simulink model "MotorCurrentEKF_"  (R2018a)
settings: Solver=VariableStepAuto  StartTime=0.0  StopTime=10.0  RelTol=1e-3
PreLoadFcn:
  | modelDir = fileparts(get_param(bdroot, 'FileName'));
  | addpath(fullfile(modelDir,'../Parameters'));
  | 
  | Parameters_Model
  | Parameters_Simulation
  | Parameters_Estimators
InitFcn:
  | Parameters_Model
  | Parameters_Simulation
  | Parameters_Estimators
undefined symbols (not defined in the file): Ke, L, P_init, X_init
settings Model: Creator=Thomas  LastModifiedBy=Thomas

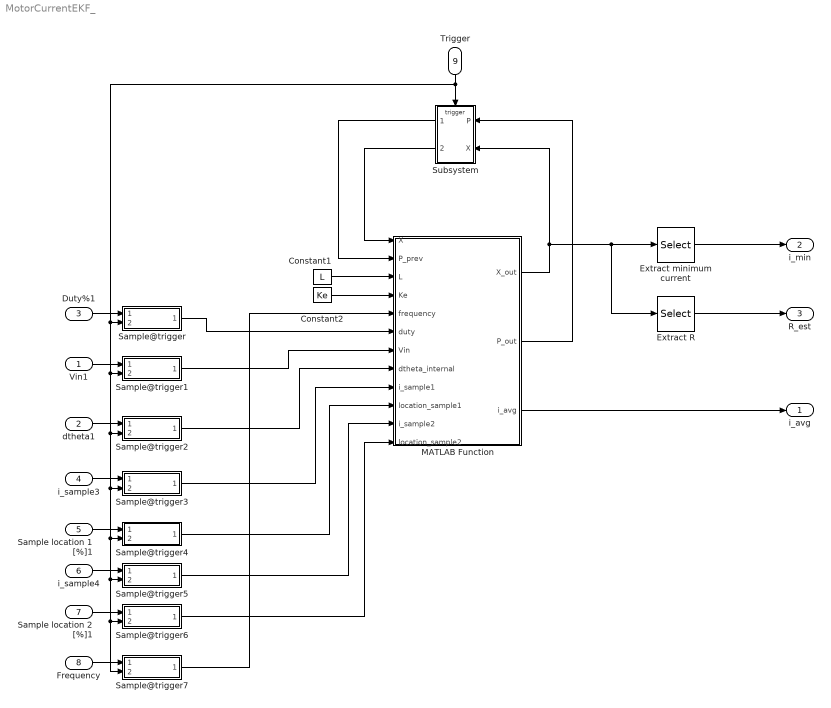
== system MotorCurrentEKF_ ==
  Vin1 : Inport  OutDataTypeStr=double
  dtheta1 : Inport  Port=2  OutDataTypeStr=double
  Duty%1 : Inport  Port=3  OutDataTypeStr=double
  i_sample3 : Inport  Port=4  OutDataTypeStr=double
  Sample location 1 [%]1 : Inport  Port=5  OutDataTypeStr=double
  i_sample4 : Inport  Port=6  OutDataTypeStr=double
  Sample location 2 [%]1 : Inport  Port=7  OutDataTypeStr=double
  Frequency : Inport  Port=8  OutDataTypeStr=double
  Trigger : Inport  Port=9  OutDataTypeStr=boolean
  Constant1 : Constant  Value=L
  Constant2 : Constant  Value=Ke
  Extract R : Selector  InputPortWidth=2  IndexOptions=Index vector (dialog)  Indices=[2]  OutputSizes=1
  Extract minimum current : Selector  InputPortWidth=2  IndexOptions=Index vector (dialog)  Indices=[1]  OutputSizes=1
  MATLAB Function : MATLAB Function  TreatAsAtomicUnit=on
  Sample@trigger : Subsystem
  Sample@trigger1 : Subsystem
  Sample@trigger2 : Subsystem
  Sample@trigger3 : Subsystem
  Sample@trigger4 : Subsystem
  Sample@trigger5 : Subsystem
  Sample@trigger6 : Subsystem
  Sample@trigger7 : Subsystem
  Subsystem : Subsystem
  i_avg : Outport
  i_min : Outport  Port=2
  R_est : Outport  Port=3
  wires:
  MATLAB Function/1(X_out) -> Subsystem/2(X), Extract R/1, Extract minimum current/1
  MATLAB Function/2(P_out) -> Subsystem/1(P)
  Subsystem/1(P_prev) -> MATLAB Function/2(P_prev)
  Subsystem/2(X_prev) -> MATLAB Function/1(X)
  Constant1/1 -> MATLAB Function/3(L)
  Constant2/1 -> MATLAB Function/4(Ke)
  MATLAB Function/3(i_avg) -> i_avg/1
  Extract minimum current/1 -> i_min/1
  Extract R/1 -> R_est/1
  Duty%1/1 -> Sample@trigger/1(Signal)
  Trigger/1 -> Sample@trigger1/2(Trigger), Sample@trigger2/2(Trigger), Sample@trigger3/2(Trigger), Sample@trigger4/2(Trigger), Sample@trigger7/2(Trigger), Sample@trigger6/2(Trigger), Sample@trigger5/2(Trigger), Sample@trigger/2(Trigger), Subsystem/Trigger
  Frequency/1 -> Sample@trigger7/1(Signal)
  Sample location 2 [%]1/1 -> Sample@trigger6/1(Signal)
  Vin1/1 -> Sample@trigger1/1(Signal)
  dtheta1/1 -> Sample@trigger2/1(Signal)
  Sample location 1 [%]1/1 -> Sample@trigger4/1(Signal)
  i_sample3/1 -> Sample@trigger3/1(Signal)
  i_sample4/1 -> Sample@trigger5/1(Signal)
  Sample@trigger/1(Sample) -> MATLAB Function/6(duty)
  Sample@trigger1/1(Sample) -> MATLAB Function/7(Vin)
  Sample@trigger2/1(Sample) -> MATLAB Function/8(dtheta_internal)
  Sample@trigger3/1(Sample) -> MATLAB Function/9(i_sample1)
  Sample@trigger4/1(Sample) -> MATLAB Function/10(location_sample1)
  Sample@trigger5/1(Sample) -> MATLAB Function/11(i_sample2)
  Sample@trigger6/1(Sample) -> MATLAB Function/12(location_sample2)
  Sample@trigger7/1(Sample) -> MATLAB Function/5(frequency)

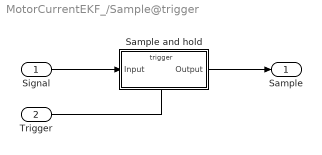
== system MotorCurrentEKF_/Sample@trigger ==
  Signal : Inport
  Trigger : Inport  Port=2
  Sample and hold : Subsystem
  Sample : Outport
  wires:
  Signal/1 -> Sample and hold/1(Input)
  Sample and hold/1(Output) -> Sample/1
  Trigger/1 -> Sample and hold/Trigger

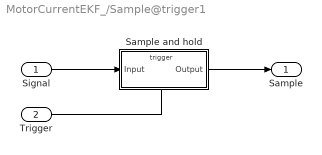
== system MotorCurrentEKF_/Sample@trigger1 ==
  Signal : Inport
  Trigger : Inport  Port=2
  Sample and hold : Subsystem
  Sample : Outport
  wires:
  Signal/1 -> Sample and hold/1(Input)
  Sample and hold/1(Output) -> Sample/1
  Trigger/1 -> Sample and hold/Trigger

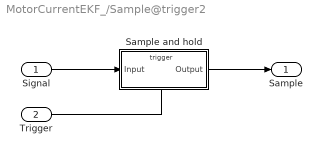
== system MotorCurrentEKF_/Sample@trigger2 ==
  Signal : Inport
  Trigger : Inport  Port=2
  Sample and hold : Subsystem
  Sample : Outport
  wires:
  Signal/1 -> Sample and hold/1(Input)
  Sample and hold/1(Output) -> Sample/1
  Trigger/1 -> Sample and hold/Trigger

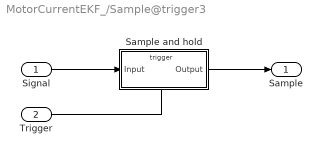
== system MotorCurrentEKF_/Sample@trigger3 ==
  Signal : Inport
  Trigger : Inport  Port=2
  Sample and hold : Subsystem
  Sample : Outport
  wires:
  Signal/1 -> Sample and hold/1(Input)
  Sample and hold/1(Output) -> Sample/1
  Trigger/1 -> Sample and hold/Trigger

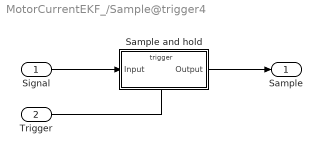
== system MotorCurrentEKF_/Sample@trigger4 ==
  Signal : Inport
  Trigger : Inport  Port=2
  Sample and hold : Subsystem
  Sample : Outport
  wires:
  Signal/1 -> Sample and hold/1(Input)
  Sample and hold/1(Output) -> Sample/1
  Trigger/1 -> Sample and hold/Trigger

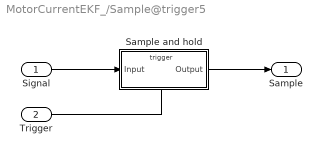
== system MotorCurrentEKF_/Sample@trigger5 ==
  Signal : Inport
  Trigger : Inport  Port=2
  Sample and hold : Subsystem
  Sample : Outport
  wires:
  Signal/1 -> Sample and hold/1(Input)
  Sample and hold/1(Output) -> Sample/1
  Trigger/1 -> Sample and hold/Trigger

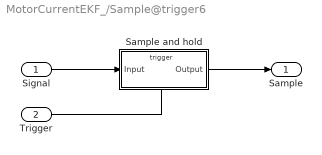
== system MotorCurrentEKF_/Sample@trigger6 ==
  Signal : Inport
  Trigger : Inport  Port=2
  Sample and hold : Subsystem
  Sample : Outport
  wires:
  Signal/1 -> Sample and hold/1(Input)
  Sample and hold/1(Output) -> Sample/1
  Trigger/1 -> Sample and hold/Trigger

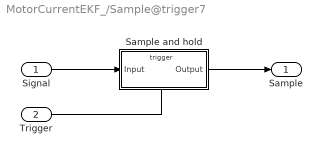
== system MotorCurrentEKF_/Sample@trigger7 ==
  Signal : Inport
  Trigger : Inport  Port=2
  Sample and hold : Subsystem
  Sample : Outport
  wires:
  Signal/1 -> Sample and hold/1(Input)
  Sample and hold/1(Output) -> Sample/1
  Trigger/1 -> Sample and hold/Trigger

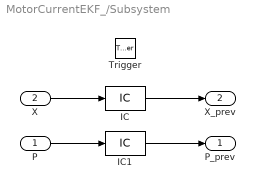
== system MotorCurrentEKF_/Subsystem ==
  P : Inport  LatchByDelayingOutsideSignal=on
  X : Inport  Port=2  LatchByDelayingOutsideSignal=on
  Trigger : TriggerPort  VariantControl=Variant  PortDimensions=1
  IC : InitialCondition  Value=X_init
  IC1 : InitialCondition  Value=P_init
  P_prev : Outport
  X_prev : Outport  Port=2
  wires:
  X/1 -> IC/1
  P/1 -> IC1/1
  IC/1 -> X_prev/1
  IC1/1 -> P_prev/1

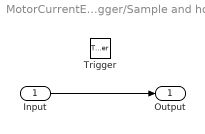
== system MotorCurrentEKF_/Sample@trigger/Sample and hold ==
  Input : Inport
  Trigger : TriggerPort  VariantControl=Variant  PortDimensions=1
  Output : Outport
  wires:
  Input/1 -> Output/1

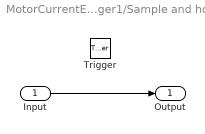
== system MotorCurrentEKF_/Sample@trigger1/Sample and hold ==
  Input : Inport
  Trigger : TriggerPort  VariantControl=Variant  PortDimensions=1
  Output : Outport
  wires:
  Input/1 -> Output/1

== system MotorCurrentEKF_/Sample@trigger2/Sample and hold ==
  Input : Inport
  Trigger : TriggerPort  VariantControl=Variant  PortDimensions=1
  Output : Outport
  wires:
  Input/1 -> Output/1

== system MotorCurrentEKF_/Sample@trigger3/Sample and hold ==
  Input : Inport
  Trigger : TriggerPort  VariantControl=Variant  PortDimensions=1
  Output : Outport
  wires:
  Input/1 -> Output/1

== system MotorCurrentEKF_/Sample@trigger4/Sample and hold ==
  Input : Inport
  Trigger : TriggerPort  VariantControl=Variant  PortDimensions=1
  Output : Outport
  wires:
  Input/1 -> Output/1

== system MotorCurrentEKF_/Sample@trigger5/Sample and hold ==
  Input : Inport
  Trigger : TriggerPort  VariantControl=Variant  PortDimensions=1
  Output : Outport
  wires:
  Input/1 -> Output/1

== system MotorCurrentEKF_/Sample@trigger6/Sample and hold ==
  Input : Inport
  Trigger : TriggerPort  VariantControl=Variant  PortDimensions=1
  Output : Outport
  wires:
  Input/1 -> Output/1

== system MotorCurrentEKF_/Sample@trigger7/Sample and hold ==
  Input : Inport
  Trigger : TriggerPort  VariantControl=Variant  PortDimensions=1
  Output : Outport
  wires:
  Input/1 -> Output/1

== matlab function MotorCurrentEKF_/MATLAB Function ==
  data: X input; X_out output; P_prev input; L input; Ke input; frequency input; duty input; Vin input; dtheta_internal input; i_sample1 input; location_sample1 input; P_out output; i_avg output; i_sample2 input; location_sample2 input
function [X_out, P_out, i_avg] = MotorCurrentEKF_(X, P_prev, ...
    L, Ke, ... % constants/parameters
    frequency, duty, Vin, dtheta_internal, ... % inputs (u)
    i_sample1, location_sample1, ...
    i_sample2, location_sample2)  % measurements (z)

%     [X_out, P_out] = MotorCurrentEKF(X, P_prev, ...
%         R, L, Ke, ... % constants/parameters
%         frequency, duty, Vin, dtheta_internal, ... % inputs (u)
%         i_meas, adc_sample_time);  % measurements (z)

    [X_out, P_out, i_avg] = MotorCurrentEKF7(X, P_prev, ...
        L, Ke, ... % constants/parameters
        frequency, duty, Vin, dtheta_internal, ... % inputs (u)
        i_sample1, location_sample1, ...
        i_sample2, location_sample2);  % measurements (z)

end
